simulink model "siso_window"  (R2021a)
settings: Solver=FixedStepDiscrete  StartTime=0.0  StopTime=1  FixedStep=1/16000  RelTol=1e-3
libraries: dspvision x1
settings Model: Creator=gonze  LastModifiedBy=chuid
settings SolverCC: AlgebraicLoopSolver=TrustRegion
settings DebuggingCC: SFMachineParentedDataDiag=warning

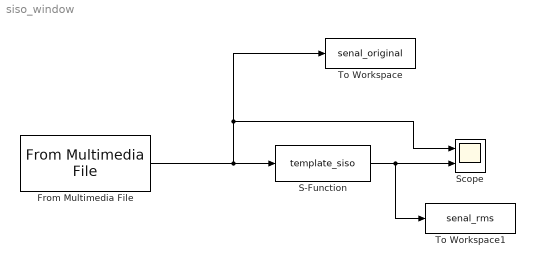
== system siso_window ==
  From Multimedia File : dspvision/From Multimedia File  inputFilename=C:\Users\chuid\Documents\GitHub\LabDSP-Repositorio\lab2dsp_G7_Aguilera_Huidobro\LabP1\scripts\musica_16_16.wav  readRange=[1 Inf]  loop=on  numPlays=inf  outputStreams=Audio only  videoDataType=single  audioDataType=double  inheritSampleTime=on  userDefinedSampleTime=1/30  noAudioOutput=off  isIntensityVideo=off  fourcc=RGB  colorVideoFormat=Separate color signals  outputEOF=off  dataOrg=Column-major  audioFrameSize=1  computeAudioFrameSize=off  outSamplingMode=Sample based
  S-Function : S-Function  FunctionName=template_siso  SFunctionDeploymentMode=off  EnableBusSupport=off
  Scope : Scope  NumInputPorts=2
  To Workspace : ToWorkspace  VariableName=senal_original  SampleTime=-1
      settings: Save2DSignal=2-D array (concatenate along first dimension)
  To Workspace1 : ToWorkspace  VariableName=senal_rms  SampleTime=-1
      settings: Save2DSignal=2-D array (concatenate along first dimension)
  wires:
  From Multimedia File/1 -> To Workspace/1, Scope/1, S-Function/1
  S-Function/1 -> To Workspace1/1, Scope/2
